simulink model "donkeycar_replay"  (R2021b)
settings: Solver=FixedStepDiscrete  StartTime=0.0  StopTime=Inf  FixedStep=0.05  RelTol=1e-3  EnableMultiTasking=on
InitFcn:
  | f=findobj('name','SDL Video Display');close(f);
libraries: matrix_library x3, deeplib x1, embedlinuxAVlib x1
settings Model: FPTRunName=Active  NumberOfSteps=10  SnapshotBufferSize=1000  ExtModeTrigDuration=2  Creator=The MathWorks, Inc.  LastModifiedBy=kkoichi
settings SolverCC: AlgebraicLoopSolver=TrustRegion  PositivePriorityOrder=on
settings DataIOCC: LimitDataPoints=on  SaveFormat=Array  SaveOutput=off  SignalLogging=off  DSMLogging=off  SaveTime=off  ReturnWorkspaceOutputs=off
settings OptimizationCC: ExpressionDepthLimit=2147483647  LifeSpan=Inf  MaxStackSize=64
settings DebuggingCC: SaveWithDisabledLinksMsg=none  SaveWithParameterizedLinksMsg=none  UnderspecifiedInitializationDetection=Classic  MergeDetectMultiDrivingBlocksExec=none  FcnCallInpInsideContextMsg=warning  AllowSymbolicDim=off  StateNameClashWarn=warning  SFUnexpectedBacktrackingDiag=warning  SFNoUnconditionalDefaultTransitionDiag=warning  SFExecutionAtInitializationDiag=none  SFMachineParentedDataDiag=warning  ArithmeticOperatorsInVariantConditions=warning
settings HardwareCC: ProdBitPerPointer=32  ProdBitPerSizeT=32  ProdBitPerPtrDiffT=32  ProdLargestAtomicInteger=Long  ProdLargestAtomicFloat=Double  ProdWordSize=32  ProdLongLongMode=on  ProdHWDeviceType=ARM Compatible->ARM Cortex  UseEmbeddedCoderFeatures=off  UseSimulinkCoderFeatures=off
settings ModelReferenceCC: PropagateSignalLabelsOutOfModel=off
settings SFSimCC: SimUseLocalCustomCode=off  CustomCodeUndefinedFunction=UseInterfaceOnly
settings RTWCC: Description=Embedded Coder  SystemTargetFile=ert.tlc  HardwareBoard=Raspberry Pi  TLCOptions="-aInlineSetEventsForThisBaseRateFcn=TLC_FALSE -aSuppressMultiTaskScheduler=TLC_FALSE  -aRateBasedStepFcn=0"  TemplateMakefile=ert_default_tmf  GenerateReport=on  RTWVerbose=off  RTWUseLocalCustomCode=off  Toolchain=GNU GCC Embedded Linux  BuildConfiguration=Faster Runs  LaunchReport=on
settings CodeAppCC: ForceParamTrailComments=on  OperatorAnnotations=on  MangleLength=10  StateflowObjectComments=on  MATLABSourceComments=on
settings ERTTargetCC: MultiwordLength=2048  ERTCustomFileBanners=off  SupportContinuousTime=on  SupportNonInlinedSFcns=on  RemoveResetFunc=off  SupportVariableSizeSignals=on  ModelStepFunctionPrototypeControlCompliant=off  ExtModeTransport=2  ExtModeStaticAlloc=on  ExtModeMexFile=ext_xcp  ExtModeIntrfLevel=Level2 - Open
settings ConfigComp: CovMetricSettings=dw  CovSaveCumulativeToWorkspaceVar=on  CovSaveSingleToWorkspaceVar=on  CovExternalEMLEnable=off  CovSFcnEnable=off

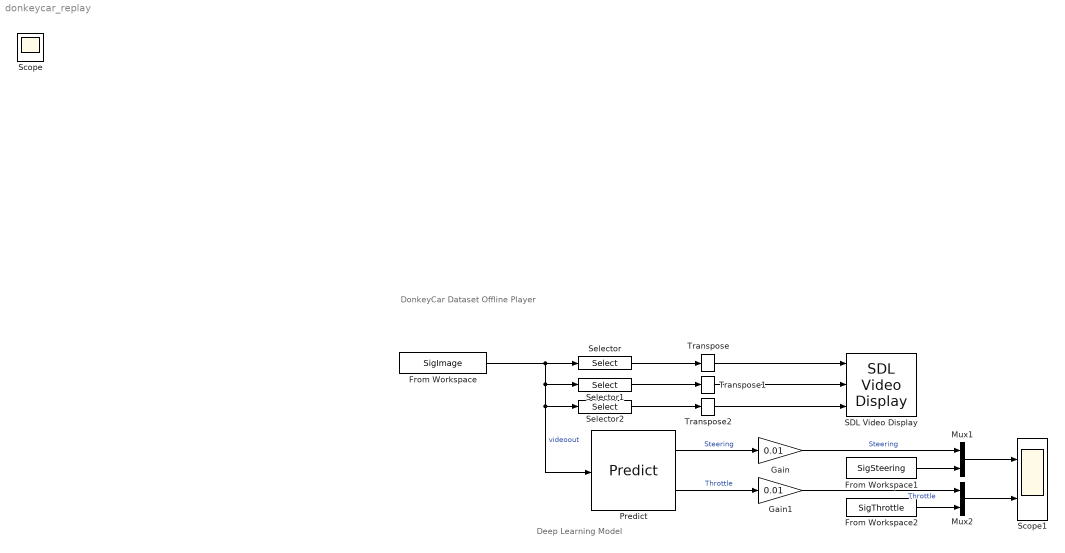
== system donkeycar_replay ==
  note: DonkeyCar Dataset Offline Player
  note: Deep Learning Model
  From Workspace : FromWorkspace  VariableName=SigImage  SampleTime=0.05
  From Workspace1 : FromWorkspace  VariableName=SigSteering  SampleTime=-1
  From Workspace2 : FromWorkspace  VariableName=SigThrottle  SampleTime=-1
  Gain : Gain  Gain=0.01  OutDataTypeStr=double
  Gain1 : Gain  Gain=0.01  OutDataTypeStr=double
  Mux1 : Mux  Inputs=2
  Mux2 : Mux  Inputs=2
  Predict : deeplib/Predict  Network=Network from MAT-file  NetworkFunction=net.mat  NetworkFilePath=donkeydata\donkeyKerasNet.mat  MiniBatchSize=128  InputDataFormats={ '', '' }  Predictions=on  Activations={}  ForceInterpretedSim=off  EnableDLNetwork=on
      settings: SourceProductBaseCode=NN
  SDL Video Display : embedlinuxAVlib/SDL Video Display  title=SDL Video Display  pixelFormat=RGB  pixelOrder=Planar  rowMajor=on  blockPlatform=Raspberry Pi
      settings: SourceProductBaseCode=SC_BEAGLEBONE_BLUE,EMBEDDEDLINUX,NVIDIA,RASPPIIO
  Scope1 : Scope  NumInputPorts=2
  Selector : Selector  NumberOfDimensions=3  InputPortWidth=3  IndexOptions=Index vector (dialog),Index vector (dialog),Index vector (dialog)  Indices=-1,-1,1  OutputSizes=1,1,1
  Selector1 : Selector  NumberOfDimensions=3  InputPortWidth=3  IndexOptions=Index vector (dialog),Index vector (dialog),Index vector (dialog)  Indices=-1,-1,2  OutputSizes=1,1,1
  Selector2 : Selector  NumberOfDimensions=3  InputPortWidth=3  IndexOptions=Index vector (dialog),Index vector (dialog),Index vector (dialog)  Indices=-1,-1,3  OutputSizes=1,1,1
  Transpose : matrix_library/Transpose
      settings: SourceProductBaseCode=SL
  Transpose1 : matrix_library/Transpose
      settings: SourceProductBaseCode=SL
  Transpose2 : matrix_library/Transpose
      settings: SourceProductBaseCode=SL
  Scope : Scope
  wires:
  Selector/1 -> Transpose/1
  Selector1/1 -> Transpose1/1
  Selector2/1 -> Transpose2/1
  Transpose/1 -> SDL Video Display/1
  Transpose1/1 -> SDL Video Display/2
  Transpose2/1 -> SDL Video Display/3
  Predict/2 -> Gain1/1  "Throttle"
  From Workspace/1 -> Predict/1, Selector2/1, Selector1/1, Selector/1  "videoout"
  Predict/1 -> Gain/1  "Steering"
  From Workspace1/1 -> Mux1/2
  Mux1/1 -> Scope1/1
  Mux2/1 -> Scope1/2
  From Workspace2/1 -> Mux2/2
  Gain/1 -> Mux1/1  "Steering"
  Gain1/1 -> Mux2/1  "Throttle"
